simulink model "LongLatDriveline"  (R2024b)
settings: Solver=FixedStepAuto  StartTime=0  StopTime=120  FixedStep=0.002  RelTol=1e-3
InitFcn:
  | load('waypoints.mat');
  | VehicleObj = Simulink.data.dictionary.open('./ModelData/VehicleData.sldd');
  | %dDataSectObj = getSection(myDictionaryObj,'Design Data');
StopFcn:
  | Plot_LateralModelErrorControl;
  | 
  | mdlWks = get_param(gcs, 'ModelWorkspace');
  | par_ToDrvDesigner = evalin(mdlWks, 'ToDrvDesigner');
  | 
  | if par_ToDrvDesigner.Value
  |     ExportdrivingScenario;
  | end
model workspace (MAT data in the model file):
  ToDrvDesigner : Simulink.Parameter (value not decoded)
values from neighbouring files (symbols this model uses):
  A_F = 2.341157    [VehicleData.sldd]
  C_af = 80000.0    [VehicleData.sldd]
  C_ar = 80000.0    [VehicleData.sldd]
  C_d = 0.24    [VehicleData.sldd]
  f = 0.01    [VehicleData.sldd]
  g = 9.81    [VehicleData.sldd]
  h_aero = 0.65    [VehicleData.sldd]
  h_gc = 0.65    [VehicleData.sldd]
  Iz = 2873.0    [VehicleData.sldd]
  lf = 1.1    [VehicleData.sldd]
  lr = 1.58    [VehicleData.sldd]
  m = 2238.932    [VehicleData.sldd]
  Nf = 2.0    [VehicleData.sldd]
  Nr = 2.0    [VehicleData.sldd]
  r_stat = 0.342    [VehicleData.sldd]
  r_w = 0.352    [VehicleData.sldd]
  rho = 1.225    [VehicleData.sldd]
  theta = 0.0    [VehicleData.sldd]
  transGear = 0.1027    [VehicleData.sldd]
  V_wind = 0.0    [VehicleData.sldd]
symbols that are objects in the model workspace (value not decoded): ToDrvDesigner
undefined symbols (not defined in the file or in its folder): InitialPsi, InitialX, InitialY, phi
libraries: slpidlib x14, spsMosfetLib x6, simulink x4, spsVoltageMeasurementLib x3, SignalEditorBlockLib x2, spsDCVoltageSourceLib x1, spspowerguiLib x1
(part 4 of 5)

== matlab function LongLatDriveline/LateralController/HOSMC_AckermanSuperTwist/HOSMC_AckermanSuperTwis1 ==
  data: U output size=1; E input; Vx input; Mu1 input; C_af parameter; g parameter; C_ar parameter; lf parameter; lr parameter; Iz parameter; m parameter; dMu1 output
% ******************* Lateral dynamic controller *********************
%*********************************************************************
% Author: L.Arturo Torres-Romero
% Date: 22-10-2020
% This controller controlls the direction of a car, based in the dynamics
% described  in the next link and using the conventional sliding mode control 
% formulation with the procedure of converting to regular form: 
% https://www.researchgate.net/publication/340166902_LATERAL_VEHICLE_DYNAMICS_AND_CONTROLLERS_DESIGN
%******************* PARAMETERS DESCRIPTIONS **********************
%******************************************************************
% m: vehicle mass
% g: gravity
% C_af : Cornering  stiffness  of  front  wheels.
% C_ar : Cornering  stiffness  of  rear  wheels.
% lf : distance fron the center of gravity to the front wheel axis.
% lr : distance fron the center of gravity to the rear wheel axis.
% Iz : this is the momentum of inertia of the vehicle respect the z axis.
%******************************************************************
%******************* INPUTS DESCRIPTIONS **************************
%******************************************************************
% E:   (column vector)[e1;de1;e2;de2] states of the state space of 
%       the system that includes the errors as follows:
%      e1  : is the lateral position error respect the road.
%      de1 : derivative of e1.
%      e2  : is the yaw angle error with respect the road. 
%      de2 : derivarive of the e2.
% Vx: Logitudinal velocity.

%******************************************************************
% ******************* OUTPUTS DESCRIPTIONS ************************
%******************************************************************
% U: control coutput in radians. Angle of the frontal wheels respect to the
%    longitudinal axis
% isCtrl: when true means that the matrix Mc has full rank, and hence, the
%         system is controllable
%******************************************************************

function [U, dMu1] = SMC_AckermanSuperTwistingCtrl(E, Vx, Mu1,C_af, g, C_ar, lf, lr, Iz, m) % pd polos deseados
X = [0; 0; 0; 0];
X(1) = E(1);
X(2) = E(2);
X(3) = E(3);
X(4) = E(4);
%**************************************************
%******* Matrix A formulation *********************
A22 = -(2*C_af + 2*C_ar)/(m*Vx);
A23 = (2*C_af + 2*C_ar)/m;
A24 = (-2*C_af*lf + 2*C_ar*lr)/(m*Vx);
A42 = -(2*C_af*lf - 2*C_ar*lr)/(Iz*Vx);
A43 = (2*C_af*lf - 2*C_ar*lr)/Iz;
A44 = -(2*C_af*lf^2 + 2*C_ar*lr^2)/(Iz*Vx);

A = [0 1 0 0;0 A22 A23 A24;0 0 0 1;0 A42 A43 A44];
%**************************************************

%**************************************************
%******* Matrix B1 formulation ********************
B1_2 = 2*C_af/m;
B1_4 = 2*C_af*lf/Iz;

B1 = [0;B1_2;0;B1_4];
%***************************************************

%***************************************************
%******* Matrix B2 formulation *********************
B2_2 = -(2*C_af*lf - 2*C_ar*lr)/(m*Vx) - Vx;
B2_4 = -(2*C_af*lf^2 + 2*C_ar*lr^2)/(Iz*Vx);

B2 = [0;B2_2;0;B2_4];
%***************************************************


%***************************************************
%******* Matrix B3 formulation *********************
B3 = [0;g;0;0];
%***************************************************


%***************************************************
%******* Verification of controllability and output 
% calculation of the controller
%**************************************************
d_k = 0;
Mc = [B1 A*B1 A^2*B1 A^3*B1];
rankVal = rank(Mc);
    if rankVal < size(A,1)
        %disp('Not completely state controllable');
        isCtrl = 0;
        d_k = 0;
    else
        %disp('Completely state controllable');
        isCtrl = 1;
        % Pole placement
        %Pd =[-5-3i -5+3i -7 -10];
        Pd =[-5-5i -5+5i -7 -10];

        H = (A- Pd(1)*eye(4)) * (A- Pd(2)*eye(4)) * (A- Pd(3)*eye(4)) * (A- Pd(4)*eye(4));

        %ackerman formula
        K = [0 0 0 1]*Mc^-1*H;
        d_k = -K*X;  
    end

%*********** Controller parameters **************
k_smc = 100;   %10
sigma = 40;    %60
gamma1 = 1;
gamma2 = 1;
gamma = [0 gamma1 0 gamma2];

h_c = gamma*[0;3;0;3];
g_c = gamma*B1;
q = 0.3;

UM = abs(h_c/g_c)/q;

%***********************************************
e_c = gamma*[0; X(1);0;X(3)];
d_u = (-1/(gamma*B1))*(sigma*sqrt(abs(e_c))*sign(e_c) + Mu1);

if abs(Mu1) > UM 
   dMu1 = -Mu1;
else
   dMu1 = -k_smc*sign(e_c); 
end

ctrlVal = d_k + d_u;

U = real(ctrlVal);

== matlab function LongLatDriveline/LateralController/SMC_ConventionalRegularForm ==
  data: U output size=1; E input; Vx input; dPsi_des input; C_af parameter; g parameter; C_ar parameter; lf parameter; lr parameter; Iz parameter; m parameter; phi_ref input

% ******************* Lateral dynamic controller *********************
%*********************************************************************
% Author: L.Arturo Torres-Romero
% Date: 22-10-2020
% This controller controlls the direction of a car, based in the dynamics
% described  in the next link and using the conventional sliding mode control 
% formulation with the procedure of converting to regular form: 
% https://www.researchgate.net/publication/340166902_LATERAL_VEHICLE_DYNAMICS_AND_CONTROLLERS_DESIGN
%******************* PARAMETERS DESCRIPTIONS **********************
%******************************************************************
% m: vehicle mass
% g: gravity
% C_af : Cornering  stiffness  of  front  wheels.
% C_ar : Cornering  stiffness  of  rear  wheels.
% lf : distance fron the center of gravity to the front wheel axis.
% lr : distance fron the center of gravity to the rear wheel axis.
% Iz : this is the momentum of inertia of the vehicle respect the z axis.
%******************************************************************
%******************* INPUTS DESCRIPTIONS **************************
%******************************************************************
% E:   (column vector)[e1;de1;e2;de2] states of the state space of 
%       the system that includes the errors as follows:
%      e1  : is the lateral position error respect the road.
%      de1 : derivative of e1.
%      e2  : is the yaw angle error with respect the road. 
%      de2 : derivarive of the e2.
% Vx: Logitudinal velocity.

%******************************************************************
% ******************* OUTPUTS DESCRIPTIONS ************************
%******************************************************************
% U: control coutput in radians. Angle of the frontal wheels respect to the
%    longitudinal axis
% isCtrl: when true means that the matrix Mc has full rank, and hence, the
%         system is controllable
%******************************************************************

function U = SMC_ConventionalCtr2(E, Vx, dPsi_des,C_af, g, C_ar, lf, lr, Iz, m, phi_ref) % pd polos deseados
J = [0; 0; 0; 0];
J(1) = E(3);
J(2) = E(4);
J(3) = E(1);
J(4) = E(2);
phi = phi_ref;
%**************************************************
%******* Matrix A formulation *********************
A22 = -(2*C_af + 2*C_ar)/(m*Vx);
A23 = (2*C_af + 2*C_ar)/m;
A24 = (-2*C_af*lf + 2*C_ar*lr)/(m*Vx);
A42 = -(2*C_af*lf - 2*C_ar*lr)/(Iz*Vx);
A43 = (2*C_af*lf - 2*C_ar*lr)/Iz;
A44 = -(2*C_af*lf^2 + 2*C_ar*lr^2)/(Iz*Vx);

%A = [0 1 0 0;0 A22 A23 A24;0 0 0 1;0 A42 A43 A44];
A = [0 0 0 1;0 A42 A43 A44;0 1 0 0;0 A22 A23 A24];

%**************************************************

%**************************************************
%******* Matrix B1 formulation ********************
B1_2 = 2*C_af/m;
B1_4 = 2*C_af*lf/Iz;

%B1 = [0;B1_2;0;B1_4];
B1 = [0;B1_4;0;B1_2];
%***************************************************

%***************************************************
%******* Matrix B2 formulation *********************
B2_2 = -(2*C_af*lf - 2*C_ar*lr)/(m*Vx) - Vx;
B2_4 = -(2*C_af*lf^2 + 2*C_ar*lr^2)/(Iz*Vx);

B2 = [0;B2_4;0;B2_2];
%***************************************************


%***************************************************
%******* Matrix B3 formulation *********************
B3 = [0;g;0;0];
%***************************************************

l1 = (A24 - Vx)*dPsi_des +g*sin(phi);
l2 = A44*dPsi_des;
L = [0;l2;0;l1];

C = [B1 A*B1 A^2*B1 A^3*B1]; % controllability matrix
Cinv = inv(C);
q = Cinv(4,:);
P = [q;q*A;q*A^2;q*A^3];
Tr = P;

X = Tr*J;

%%%%%%%%%%%%%%%%%%%%%%%%%%%%% SMC settings %%%%%%%%%%%%%%%%%%%%%%%%%%%%%%%
n1 = 140000;
lambda_1 = -2;
lambda_2 = -7;
lambda_3 = -3;

S = [(1000000*lambda_1*lambda_2*lambda_3)/(A23*B1_4 - A43*B1_2), (1000000*(A23^2*B1_4^3 + A43^2*B1_2^2*B1_4 + A22*A23*A24*B1_4^3 - A42*A43*A44*B1_2^3 - 2*A23*A43*B1_2*B1_4^2 - A43*A44*B1_2^3*lambda_1 - A43*A44*B1_2^3*lambda_2 - A43*A44*B1_2^3*lambda_3 - A22*A23*A44*B1_2*B1_4^2 - A22*A24*A43*B1_2*B1_4^2 - A23*A24*A42*B1_2*B1_4^2 + A22*A43*A44*B1_2^2*B1_4 + A23*A42*A44*B1_2^2*B1_4 + A24*A42*A43*B1_2^2*B1_4 - A23*A24*B1_2*B1_4^2*lambda_1 - A23*A24*B1_2*B1_4^2*lambda_2 - A23*A24*B1_2*B1_4^2*lambda_3 + A23*A44*B1_2^2*B1_4*lambda_1 + A24*A43*B1_2^2*B1_4*lambda_1 + A23*A44*B1_2^2*B1_4*lambda_2 + A24*A43*B1_2^2*B1_4*lambda_2 + A23*A44*B1_2^2*B1_4*lambda_3 + A24*A43*B1_2^2*B1_4*lambda_3 - A23*B1_2*B1_4^2*lambda_1*lambda_2 - A23*B1_2*B1_4^2*lambda_1*lambda_3 - A23*B1_2*B1_4^2*lambda_2*lambda_3 + A43*B1_2^2*B1_4*lambda_1*lambda_2 + A43*B1_2^2*B1_4*lambda_1*lambda_3 + A43*B1_2^2*B1_4*lambda_2*lambda_3 - A44*B1_2^3*lambda_1*lambda_2*lambda_3 + A22*B1_2*B1_4^2*lambda_1*lambda_2*lambda_3 + A24*B1_2^2*B1_4*lambda_1*lambda_2*lambda_3 - A42*B1_2^2*B1_4*lambda_1*lambda_2*lambda_3))/((A23*B1_4 - A43*B1_2)*(A24^2*B1_2*B1_4^2 - 2*A24*A44*B1_2^2*B1_4 - A42*A24*B1_2*B1_4^2 + A22*A24*B1_4^3 + A44^2*B1_2^3 + A42*A44*B1_2^2*B1_4 - A22*A44*B1_2*B1_4^2 - A43*B1_2*B1_4^2 + A23*B1_4^3)), (1000000*(A23^2*B1_4^3*lambda_1 + A23^2*B1_4^3*lambda_2 + A23^2*B1_4^3*lambda_3 + A23^2*A24*B1_4^3 - A43^2*A44*B1_2^3 + A24*A43^2*B1_2^2*B1_4 - A23^2*A44*B1_2*B1_4^2 + A43^2*B1_2^2*B1_4*lambda_1 + A43^2*B1_2^2*B1_4*lambda_2 + A43^2*B1_2^2*B1_4*lambda_3 - 2*A23*A24*A43*B1_2*B1_4^2 + 2*A23*A43*A44*B1_2^2*B1_4 - 2*A23*A43*B1_2*B1_4^2*lambda_1 - 2*A23*A43*B1_2*B1_4^2*lambda_2 - 2*A23*A43*B1_2*B1_4^2*lambda_3 - A22*A23*B1_4^3*lambda_1*lambda_2 - A22*A23*B1_4^3*lambda_1*lambda_3 - A22*A23*B1_4^3*lambda_2*lambda_3 - A43*A44*B1_2^3*lambda_1*lambda_2 - A43*A44*B1_2^3*lambda_1*lambda_3 - A43*A44*B1_2^3*lambda_2*lambda_3 + A22^2*B1_4^3*lambda_1*lambda_2*lambda_3 + A42^2*B1_2^2*B1_4*lambda_1*lambda_2*lambda_3 - A23*A24*B1_2*B1_4^2*lambda_1*lambda_2 - A23*A24*B1_2*B1_4^2*lambda_1*lambda_3 - A23*A24*B1_2*B1_4^2*lambda_2*lambda_3 + A22*A43*B1_2*B1_4^2*lambda_1*lambda_2 + A23*A42*B1_2*B1_4^2*lambda_1*lambda_2 + A22*A43*B1_2*B1_4^2*lambda_1*lambda_3 + A23*A42*B1_2*B1_4^2*lambda_1*lambda_3 + A22*A43*B1_2*B1_4^2*lambda_2*lambda_3 + A23*A42*B1_2*B1_4^2*lambda_2*lambda_3 + A23*A44*B1_2^2*B1_4*lambda_1*lambda_2 + A24*A43*B1_2^2*B1_4*lambda_1*lambda_2 + A23*A44*B1_2^2*B1_4*lambda_1*lambda_3 + A24*A43*B1_2^2*B1_4*lambda_1*lambda_3 + A23*A44*B1_2^2*B1_4*lambda_2*lambda_3 + A24*A43*B1_2^2*B1_4*lambda_2*lambda_3 - A42*A43*B1_2^2*B1_4*lambda_1*lambda_2 - A42*A43*B1_2^2*B1_4*lambda_1*lambda_3 - A42*A43*B1_2^2*B1_4*lambda_2*lambda_3 + A42*A44*B1_2^3*lambda_1*lambda_2*lambda_3 - A23*B1_2*B1_4^2*lambda_1*lambda_2*lambda_3 + A43*B1_2^2*B1_4*lambda_1*lambda_2*lambda_3 + A22*A24*B1_2*B1_4^2*lambda_1*lambda_2*lambda_3 - 2*A22*A42*B1_2*B1_4^2*lambda_1*lambda_2*lambda_3 - A22*A44*B1_2^2*B1_4*lambda_1*lambda_2*lambda_3 - A24*A42*B1_2^2*B1_4*lambda_1*lambda_2*lambda_3))/((A23*B1_4 - A43*B1_2)*(A24^2*B1_2*B1_4^2 - 2*A24*A44*B1_2^2*B1_4 - A42*A24*B1_2*B1_4^2 + A22*A24*B1_4^3 + A44^2*B1_2^3 + A42*A44*B1_2^2*B1_4 - A22*A44*B1_2*B1_4^2 - A43*B1_2*B1_4^2 + A23*B1_4^3)), (1000000*(A23*A24^2*B1_4^3 - A43*A44^2*B1_2^3 + A23*B1_4^3*lambda_1*lambda_2 + A23*B1_4^3*lambda_1*lambda_3 + A23*B1_4^3*lambda_2*lambda_3 + A23*A44^2*B1_2^2*B1_4 - A24^2*A43*B1_2*B1_4^2 + A23*A24*B1_4^3*lambda_1 + A23*A24*B1_4^3*lambda_2 + A23*A24*B1_4^3*lambda_3 - 2*A23*A24*A44*B1_2*B1_4^2 + 2*A24*A43*A44*B1_2^2*B1_4 - A23*A44*B1_2*B1_4^2*lambda_1 - A24*A43*B1_2*B1_4^2*lambda_1 - A23*A44*B1_2*B1_4^2*lambda_2 - A24*A43*B1_2*B1_4^2*lambda_2 - A23*A44*B1_2*B1_4^2*lambda_3 - A24*A43*B1_2*B1_4^2*lambda_3 + A43*A44*B1_2^2*B1_4*lambda_1 + A43*A44*B1_2^2*B1_4*lambda_2 + A43*A44*B1_2^2*B1_4*lambda_3 - A43*B1_2*B1_4^2*lambda_1*lambda_2 - A43*B1_2*B1_4^2*lambda_1*lambda_3 - A43*B1_2*B1_4^2*lambda_2*lambda_3 - A22*B1_4^3*lambda_1*lambda_2*lambda_3 - A24*B1_2*B1_4^2*lambda_1*lambda_2*lambda_3 + A42*B1_2*B1_4^2*lambda_1*lambda_2*lambda_3 + A44*B1_2^2*B1_4*lambda_1*lambda_2*lambda_3))/((A23*B1_4 - A43*B1_2)*(A24^2*B1_2*B1_4^2 - 2*A24*A44*B1_2^2*B1_4 - A42*A24*B1_2*B1_4^2 + A22*A24*B1_4^3 + A44^2*B1_2^3 + A42*A44*B1_2^2*B1_4 - A22*A44*B1_2*B1_4^2 - A43*B1_2*B1_4^2 + A23*B1_4^3))];

%%%%%%%%%%%%%%%%%%%%%%%%%%%%%%%%%%%%%%%%%%%%%%%%%%%%%%%%%%%%%%%%%%%%%%%%%%%%

sigma1 = S*X;
ctrlVal = -(S*B1)\(n1*sign(sigma1)+ S*A*X +S*L);
U = real(ctrlVal);    



%*****************************************************************************
%******* Live script for help in calculus of the controller ************
% 
% format rational
% syms A B Q R Tr B1_2 B1_4 A22 A23 A24 A42 A43 A44 delta x1 x2 x3 x4 l1 l2
% 
% % X  = [x1;x2;x3;x4]
% % A  = [0 1 0 0;0 A22 A23 A24;0 0 0 1;0 A42 A43 A44]
% % B1 = [0;B1_2;0;B1_4]
% % L  = [0;l1;0;l2]
% 
% X  = [x3;x4;x1;x2]
% A  = [0 0 0 1;0 A42 A43 A44;0 1 0 0;0 A22 A23 A24]
% B1 = [0;B1_4;0;B1_2]
% L  = [0;l2;0;l1]
% 
% %%%%%%%%%%%%%%%% Transform (Tr) with ackerman form %%%%%%%%%%%%%%%%
% % C = [B1 A*B1 A^2*B1 A^3*B1] % controllability matrix
% % tmp1 = [0 0 0 1]/C;
% % Tr=[tmp1;tmp1*A;tmp1*A^2;tmp1*A^3] % state transformation
% % disp("tmp1")
% % size(tmp1)
% % disp("tmp1*A")
% % size(tmp1*A)
% % disp("tmp1*A^2")
% % size(tmp1*A^2)
% % disp("tmp1*A^3")
% % size(tmp1*A^3)
% % disp("C:")
% % size(C)
% % disp("tmp1:")
% % size(tmp1)
% % disp("Tr:")
% % size(Tr)
% %%%%%%%%%%%%%%%%%%%%%%%%%%%%%%%%%%%%%%%%%%%%%%%%%%%%%%%%%%%%%%%%%
% 
% %%%%%%%%%%%% Transform (Tr) with Utkin apprach %%%%%%%%%%%%%%%%%%
% % B_1 = [0;0;B1_4];
% % B_2 = B1_2;
% % 
% % a = eye(3)
% % b = -B_1*(B_2^(-1))
% % c = [0 0 0]
% % d = B_2^(-1)
% % 
% % Tr = [a b;c d];
% %%%%%%%%%%%%%%%%%%%%%%%%%%%%%%%%%%%%%%%%%%%%%%%%%%%%%%%%%%%%%%%%%%
% 
% 
% %%%%%%%%%%%%%%%% Transform (Tr) with linear system controller form %%%%%%%%%%%%%%%%
% C = [B1 A*B1 A^2*B1 A^3*B1] % controllability matrix
% Cinv = inv(C)
% q = Cinv(4,:)
% P = [q;q*A;q*A^2;q*A^3]
% Tr = P
% %%%%%%%%%%%%%%%%%%%%%%%%%%%%%%%%%%%%%%%%%%%%%%%%%%%%%%%%%%
% 
% A_ = simplify(Tr*A/Tr)
% B_ = simplify(Tr*B1)
% 
% A_11 = A_(1:3,1:3);
% A_12 = A_(1:3,4);
% 
% syms s1 s2 s3 lambda lambda_1 lambda_2 lambda_3 S2
% 
% %find paramters given eigenvalues
% S = [s1 s2 s3];
% eqeigen = det(lambda*eye(3) - (A_11 - A_12*S));
% eqeigen = simplify(eqeigen);
% eqeigen = collect(eqeigen,lambda);
% polyCoef = coeffs(eqeigen, lambda);
% polyCoef = fliplr(polyCoef)
% %%%%%%%%%%%%%%%
% % desired polinomial characteristic
% desiredPoly = (lambda + lambda_1)*(lambda + lambda_2)*(lambda + lambda_3);
% desiredPoly = collect(desiredPoly);
% desiredCoefs = coeffs(desiredPoly, lambda);
% desiredCoefs = fliplr(desiredCoefs)
% 
% eq1 = desiredCoefs(1) == polyCoef(1);
% eq2 = desiredCoefs(2) == polyCoef(2);
% eq3 = desiredCoefs(3) == polyCoef(3);
% eq4 = desiredCoefs(4) == polyCoef(4);
% 
% system1 = [eq2;eq3;eq4];
% sol = solve(system1,[s1 s2 s3]);
% S_ = [sol.s1 sol.s2 sol.s3]
% 
% %test eigen values:
% charEq1 = subs(eqeigen,s1,sol.s1);
% charEq2 = subs(charEq1,s2,sol.s2);
% charEq3 = subs(charEq2,s3,sol.s3)
% tf = isAlways(charEq3==desiredPoly)
% 
% S2 = 1000000;
% S = S2*[S_ 1]*Tr;
% %S = [S_ 1]*Tr;
% disp("!!!!!!!!surface S: ")
% simplify(S)
% 
% 
% syms n sigma1 x1 x2 x3 x4 u1 u2 n1 n2 
% X = [x1;x2;x3;x4];
% U = u1;
% 
% SIGMA = S*X;
% 
% % rewriting to the original forms %%%%%%%%%%%%%%%
% X  = [x1;x2;x3;x4]
% A  = [0 1 0 0;0 A22 A23 A24;0 0 0 1;0 A42 A43 A44]
% B1 = [0;B1_2;0;B1_4]
% %%%%%%%%%%%%%%%%%%%%%%%%%%%%%%%%%%%%%%%%%%%%%%%
% 
% 
% disp("!!!!! Sliding function sigma_1: ")
% Sigma_1 = simplify(SIGMA);
% Sigma_1 = collect(Sigma_1,[x1;x2;x3;x4])
% 
% eqsolution = -n1*sign(sigma1) == S*(A*X + B1*U +L);
% sol1 = solve(eqsolution,u1);
% 
% disp("!!!!! final control u: ")
% finalControl = simplify(sol1);
% finalControl = collect(finalControl,[x1;x2;x3;x4])
% 
% 
% U = -inv(S*B1)*(n1*sign(sigma1)+ S*A*X +S*L)
% 
% isAlways(finalControl==U)

== matlab function LongLatDriveline/Power Module/BLDC Motor/BLDC  SVPWM/Fases abc1 ==
  data: X input; Fabc output
function Fabc = fcn(X)
Fabc = [0;0;0];
    theta = mod(X(4),2*pi); %X(4)
    %theta = mod(X,2*pi);
    
    if (0<=theta)&&(theta<(pi/6))
        Fa = (6/pi)*theta;
    elseif ((pi/6)<=theta)&&(theta<(5*pi/6))
        Fa = 1;
    elseif ((5*pi/6<=theta))&&(theta<(7*pi/6))
        Fa = (6/pi)*(pi-theta);
    elseif ((7*pi/6)<=theta)&&(theta<(11*pi/6))
        Fa = -1;
    elseif ((11*pi/6)<=theta)&&(theta<(2*pi))
        Fa = (6/pi)*(theta-2*pi);
    else
        Fa = NaN;
    end
    
    if (0<=theta)&&(theta<(3*pi/6))
        Fb = -1;
    elseif ((3*pi/6)<=theta)&&(theta<(5*pi/6))
        Fb = (6/pi)*(theta-(2*pi)/3);
    elseif ((5*pi/6)<=theta)&&(theta<(9*pi/6))
        Fb = 1;
    elseif ((9*pi/6)<=theta)&&(theta<(11*pi/6))
        Fb = (6/pi)*(-theta+(5*pi)/3);
    elseif ((11*pi/6)<=theta)&&(theta<(2*pi))
        Fb = -1;
    else
        Fb = NaN;
    end
    
    if (0<=theta)&&(theta<(pi/6))
        Fc = 1;
    elseif ((pi/6)<=theta)&&(theta<(3*pi/6))
        Fc = (6/pi)*(pi/3-theta);
    elseif ((3*pi/6)<=theta)&&(theta<(7*pi/6))
        Fc = -1;
    elseif ((7*pi/6)<=theta)&&(theta<(9*pi/6))
        Fc = (6/pi)*(theta-(4*pi)/3);
    elseif ((9*pi/6)<=theta)&&(theta<(2*pi))
        Fc = 1;
    else
        Fc = NaN; 
    end
    
    
%     
     Fa = sin(theta);
     Fb = sin(theta - 2*pi/3);
     Fc = sin(theta + 2*pi/3);
    
    Fabc = [Fa;Fb;Fc];
end

== matlab function LongLatDriveline/LateralController/HOSMC_IntegralBlocksSuperTwisting/HOSMC_SuperTwisting ==
  data: U output size=1; d_k output; d_u output; E input; Vx input; dPsi_des input; phi_ref input; v input; e_bn input; C_af parameter; g parameter; C_ar parameter; lf parameter; lr parameter; Iz parameter; m parameter; dv output; de_bn output
% ******************* Lateral dynamic controller *********************

%*********************************************************************
% Author: L.Arturo Torres-Romero
% Date: 22-10-2025
% This controller controlls the direction of a car, based in the dynamics
% of the control by blocks with integral super-twisting SMC.
%  
% 
%******************* PARAMETERS DESCRIPTIONS **********************
%******************************************************************
% m: vehicle mass
% g: gravity
% C_af : Cornering  stiffness  of  front  wheels.
% C_ar : Cornering  stiffness  of  rear  wheels.
% lf : distance fron the center of gravity to the front wheel axis.
% lr : distance fron the center of gravity to the rear wheel axis.
% Iz : this is the momentum of inertia of the vehicle respect the z axis.
%******************************************************************
%******************* INPUTS DESCRIPTIONS **************************
%******************************************************************
% E:   (column vector)[e1;de1;e2;de2] states of the state space of 
%       the system that includes the errors as follows:
%      e1  : is the lateral position error respect the road.
%      de1 : derivative of e1.
%      e2  : is the yaw angle error with respect the road. 
%      de2 : derivarive of the e2.
% Vx: Logitudinal velocity.
% dPsi_des : Yaw derivative according the actual speed and road.
% phi_ref  : Superelevation of the road defined in the waipoints file. 
% v        : Integrated part of the STA.
% e_bn     : Nominal response of the error.
%******************************************************************
% ******************* OUTPUTS DESCRIPTIONS ************************
%******************************************************************
% U: control coutput in radians. Angle of the frontal wheels respect to the
%    longitudinal axis.
% d_k: Linear part of the control based on the known terms.
% d_u: Non linear part of the control bases on SMC super-twisting.
% dv : Switching part of the STA.
% de_bn: Dynamic of the nominal error.
%******************************************************************
function [U, d_k,d_u,dv,de_bn] = HOSMC_SuperTwistingCtrl...
    (E, Vx,dPsi_des, phi_ref, v,e_bn, C_af, g, C_ar, lf, lr, Iz, m) 
Y1 = [0;0];
Y2 = [0;0];

Y1 = [E(1);E(3)];
Y2 = [E(2);E(4)];
e = [E(2);E(3);E(4)];
%en = [Y2n(1); Y1n(2); Y2n(2)];
phi = phi_ref;

%**************************************************
%******* Matrix A formulation *********************
A22 = -(2*C_af + 2*C_ar)/(m*Vx);
A23 = (2*C_af + 2*C_ar)/m;
A24 = (-2*C_af*lf + 2*C_ar*lr)/(m*Vx);
A42 = -(2*C_af*lf - 2*C_ar*lr)/(Iz*Vx);
A43 = (2*C_af*lf - 2*C_ar*lr)/Iz;
A44 = -(2*C_af*lf^2 + 2*C_ar*lr^2)/(Iz*Vx);

A = [A22 A23 A24;A42 A43 A44];

%**************************************************
%******* Matrix B1 formulation ********************
B1_2 = 2*C_af/m;
B1_4 = 2*C_af*lf/Iz;

B1 = [B1_2;B1_4];
%***************************************************

%***************************************************
%******* Matrix L formulation *********************
l1 = (A24 - Vx)*dPsi_des +g*sin(phi);
l2 = A44*dPsi_des;
L = [l1;l2];

%***************************************************

%%
%%%%%%%%%%%%%% SUPER TWISTING 1 %%%%%%%%%%%%%%%%%
% %*********** Controller parameters **************
% k1 = 1;%6;      %7   18
% k2 = 15;%8;
%sigma = 10;    %60   10
gamma1 = 5;
gamma2 = 1;
gamma = [gamma1 gamma2];
%***************************************
h_c = abs(gamma*[0.8;0.4]);
g_c = abs(gamma*B1);
U_M = pi/8;

q = abs(h_c/g_c)/U_M;
C = abs(h_c);
k_v = C/(gamma*B1); %k_v = C/(gamma*B1) + 0.5;

k_u = sqrt(2/(gamma*B1*k_v - C));
k_u = k_u*(gamma*B1*k_v + C)*(1+q);
k_u = k_u/((gamma*B1)*(1-q)); %k_u = k_u/((gamma*B1)*(1-q)) + 0.8;


%*** Gains for s1 *******
k_v = 0.0065*1;
k_u = 0.0012*1.3;
%**********************


%***********************************************
k1 = 9;% 13.5
k2 = 8;% 5
e_b = -gamma*(k1*Y1+Y2);
d_k = -(1/(gamma*B1))*(gamma*(k1*Y2+A*e+L)-k2*e_b);

% dY2n = A*e + B1*d_k + L;
% dY1n = Y2n;


%************ two options for SMC surfaces *******
de_bn = -gamma*(k1*Y2 + A*e + B1*d_k + L);
s1 =  k2*(e_bn-e_b);


%***** the integration of dY1, dY2 must be implemented for this option
% e_t = gamma*(k1*Y1+Y2);     
% e_tn = gamma*(k1*Y1n+Y2n);
%s2 = e_t - e_tn; %(surface over the whole error of the states)
%*************************************************

s = s1;

d_u = -k_u*sqrt(abs(s))*sign(s) + v;

if abs(d_u) > U_M 
   dv = -d_u;
else
   dv = -k_v*sign(s); 
end

%%

%ctrlVal = d_k;
ctrlVal = d_k + d_u;
U = real(ctrlVal);

== matlab function LongLatDriveline/LateralController/HOSMC_RegularFormSuperTwist/HOSMC_RegularFormSuperTwist ==
  data: U output size=1; E input; Vx input; dPsi_des input; Mu1 input; C_af parameter; g parameter; C_ar parameter; lf parameter; lr parameter; Iz parameter; m parameter; dMu1 output; phi parameter
% ******************* Lateral dynamic controller *********************

%*********************************************************************
% Author: L.Arturo Torres-Romero
% Date: 22-10-2020
% This controller controlls the direction of a car, based in the dynamics
% described  in the next link and using the conventional sliding mode control 
% formulation with the procedure of converting to regular form: 
% https://www.researchgate.net/publication/340166902_LATERAL_VEHICLE_DYNAMICS_AND_CONTROLLERS_DESIGN
%******************* PARAMETERS DESCRIPTIONS **********************
%******************************************************************
% m: vehicle mass
% g: gravity
% C_af : Cornering  stiffness  of  front  wheels.
% C_ar : Cornering  stiffness  of  rear  wheels.
% lf : distance fron the center of gravity to the front wheel axis.
% lr : distance fron the center of gravity to the rear wheel axis.
% Iz : this is the momentum of inertia of the vehicle respect the z axis.
%******************************************************************
%******************* INPUTS DESCRIPTIONS **************************
%******************************************************************
% E:   (column vector)[e1;de1;e2;de2] states of the state space of 
%       the system that includes the errors as follows:
%      e1  : is the lateral position error respect the road.
%      de1 : derivative of e1.
%      e2  : is the yaw angle error with respect the road. 
%      de2 : derivarive of the e2.
% Vx: Logitudinal velocity.

%******************************************************************
% ******************* OUTPUTS DESCRIPTIONS ************************
%******************************************************************
% U: control coutput in radians. Angle of the frontal wheels respect to the
%    longitudinal axis
% isCtrl: when true means that the matrix Mc has full rank, and hence, the
%         system is controllable
%******************************************************************

function [U, dMu1] = HOSMC_RegularFormSuperTwistCtrl(E, Vx,dPsi_des, Mu1,C_af, g, C_ar, lf, lr, Iz, m,phi) % pd polos deseados
J = [0; 0; 0; 0];
J(1) = E(3);
J(2) = E(4);
J(3) = E(1);
J(4) = E(2);

%**************************************************
%******* Matrix A formulation *********************
A22 = -(2*C_af + 2*C_ar)/(m*Vx);
A23 = (2*C_af + 2*C_ar)/m;
A24 = (-2*C_af*lf + 2*C_ar*lr)/(m*Vx);
A42 = -(2*C_af*lf - 2*C_ar*lr)/(Iz*Vx);
A43 = (2*C_af*lf - 2*C_ar*lr)/Iz;
A44 = -(2*C_af*lf^2 + 2*C_ar*lr^2)/(Iz*Vx);

%A = [0 1 0 0;0 A22 A23 A24;0 0 0 1;0 A42 A43 A44];
A = [0 0 0 1;0 A42 A43 A44;0 1 0 0;0 A22 A23 A24];

%**************************************************

%**************************************************
%******* Matrix B1 formulation ********************
B1_2 = 2*C_af/m;
B1_4 = 2*C_af*lf/Iz;

%B1 = [0;B1_2;0;B1_4];
B1 = [0;B1_4;0;B1_2];
%***************************************************

%***************************************************
%******* Matrix B2 formulation *********************
B2_2 = -(2*C_af*lf - 2*C_ar*lr)/(m*Vx) - Vx;
B2_4 = -(2*C_af*lf^2 + 2*C_ar*lr^2)/(Iz*Vx);

B2 = [0;B2_4;0;B2_2];
%***************************************************


%***************************************************
%******* Matrix B3 formulation *********************
B3 = [0;g;0;0];
%***************************************************

l1 = (A24 - Vx)*dPsi_des +g*sin(phi);
l2 = A44*dPsi_des;
L = [0;l2;0;l1];

C = [B1 A*B1 A^2*B1 A^3*B1]; % controllability matrix
Cinv = inv(C);
q = Cinv(4,:);
P = [q;q*A;q*A^2;q*A^3];
Tr = P;

X = Tr*J;

%%%%%%%%%%%%%%%%%%%%%%%%%%%%% SMC settings %%%%%%%%%%%%%%%%%%%%%%%%%%%%%%%
n1 = 1;%140000;
lambda_1 = -2;
lambda_2 = -7;
lambda_3 = -3;

S = [(1000000*lambda_1*lambda_2*lambda_3)/(A23*B1_4 - A43*B1_2), (1000000*(A23^2*B1_4^3 + A43^2*B1_2^2*B1_4 + A22*A23*A24*B1_4^3 - A42*A43*A44*B1_2^3 - 2*A23*A43*B1_2*B1_4^2 - A43*A44*B1_2^3*lambda_1 - A43*A44*B1_2^3*lambda_2 - A43*A44*B1_2^3*lambda_3 - A22*A23*A44*B1_2*B1_4^2 - A22*A24*A43*B1_2*B1_4^2 - A23*A24*A42*B1_2*B1_4^2 + A22*A43*A44*B1_2^2*B1_4 + A23*A42*A44*B1_2^2*B1_4 + A24*A42*A43*B1_2^2*B1_4 - A23*A24*B1_2*B1_4^2*lambda_1 - A23*A24*B1_2*B1_4^2*lambda_2 - A23*A24*B1_2*B1_4^2*lambda_3 + A23*A44*B1_2^2*B1_4*lambda_1 + A24*A43*B1_2^2*B1_4*lambda_1 + A23*A44*B1_2^2*B1_4*lambda_2 + A24*A43*B1_2^2*B1_4*lambda_2 + A23*A44*B1_2^2*B1_4*lambda_3 + A24*A43*B1_2^2*B1_4*lambda_3 - A23*B1_2*B1_4^2*lambda_1*lambda_2 - A23*B1_2*B1_4^2*lambda_1*lambda_3 - A23*B1_2*B1_4^2*lambda_2*lambda_3 + A43*B1_2^2*B1_4*lambda_1*lambda_2 + A43*B1_2^2*B1_4*lambda_1*lambda_3 + A43*B1_2^2*B1_4*lambda_2*lambda_3 - A44*B1_2^3*lambda_1*lambda_2*lambda_3 + A22*B1_2*B1_4^2*lambda_1*lambda_2*lambda_3 + A24*B1_2^2*B1_4*lambda_1*lambda_2*lambda_3 - A42*B1_2^2*B1_4*lambda_1*lambda_2*lambda_3))/((A23*B1_4 - A43*B1_2)*(A24^2*B1_2*B1_4^2 - 2*A24*A44*B1_2^2*B1_4 - A42*A24*B1_2*B1_4^2 + A22*A24*B1_4^3 + A44^2*B1_2^3 + A42*A44*B1_2^2*B1_4 - A22*A44*B1_2*B1_4^2 - A43*B1_2*B1_4^2 + A23*B1_4^3)), (1000000*(A23^2*B1_4^3*lambda_1 + A23^2*B1_4^3*lambda_2 + A23^2*B1_4^3*lambda_3 + A23^2*A24*B1_4^3 - A43^2*A44*B1_2^3 + A24*A43^2*B1_2^2*B1_4 - A23^2*A44*B1_2*B1_4^2 + A43^2*B1_2^2*B1_4*lambda_1 + A43^2*B1_2^2*B1_4*lambda_2 + A43^2*B1_2^2*B1_4*lambda_3 - 2*A23*A24*A43*B1_2*B1_4^2 + 2*A23*A43*A44*B1_2^2*B1_4 - 2*A23*A43*B1_2*B1_4^2*lambda_1 - 2*A23*A43*B1_2*B1_4^2*lambda_2 - 2*A23*A43*B1_2*B1_4^2*lambda_3 - A22*A23*B1_4^3*lambda_1*lambda_2 - A22*A23*B1_4^3*lambda_1*lambda_3 - A22*A23*B1_4^3*lambda_2*lambda_3 - A43*A44*B1_2^3*lambda_1*lambda_2 - A43*A44*B1_2^3*lambda_1*lambda_3 - A43*A44*B1_2^3*lambda_2*lambda_3 + A22^2*B1_4^3*lambda_1*lambda_2*lambda_3 + A42^2*B1_2^2*B1_4*lambda_1*lambda_2*lambda_3 - A23*A24*B1_2*B1_4^2*lambda_1*lambda_2 - A23*A24*B1_2*B1_4^2*lambda_1*lambda_3 - A23*A24*B1_2*B1_4^2*lambda_2*lambda_3 + A22*A43*B1_2*B1_4^2*lambda_1*lambda_2 + A23*A42*B1_2*B1_4^2*lambda_1*lambda_2 + A22*A43*B1_2*B1_4^2*lambda_1*lambda_3 + A23*A42*B1_2*B1_4^2*lambda_1*lambda_3 + A22*A43*B1_2*B1_4^2*lambda_2*lambda_3 + A23*A42*B1_2*B1_4^2*lambda_2*lambda_3 + A23*A44*B1_2^2*B1_4*lambda_1*lambda_2 + A24*A43*B1_2^2*B1_4*lambda_1*lambda_2 + A23*A44*B1_2^2*B1_4*lambda_1*lambda_3 + A24*A43*B1_2^2*B1_4*lambda_1*lambda_3 + A23*A44*B1_2^2*B1_4*lambda_2*lambda_3 + A24*A43*B1_2^2*B1_4*lambda_2*lambda_3 - A42*A43*B1_2^2*B1_4*lambda_1*lambda_2 - A42*A43*B1_2^2*B1_4*lambda_1*lambda_3 - A42*A43*B1_2^2*B1_4*lambda_2*lambda_3 + A42*A44*B1_2^3*lambda_1*lambda_2*lambda_3 - A23*B1_2*B1_4^2*lambda_1*lambda_2*lambda_3 + A43*B1_2^2*B1_4*lambda_1*lambda_2*lambda_3 + A22*A24*B1_2*B1_4^2*lambda_1*lambda_2*lambda_3 - 2*A22*A42*B1_2*B1_4^2*lambda_1*lambda_2*lambda_3 - A22*A44*B1_2^2*B1_4*lambda_1*lambda_2*lambda_3 - A24*A42*B1_2^2*B1_4*lambda_1*lambda_2*lambda_3))/((A23*B1_4 - A43*B1_2)*(A24^2*B1_2*B1_4^2 - 2*A24*A44*B1_2^2*B1_4 - A42*A24*B1_2*B1_4^2 + A22*A24*B1_4^3 + A44^2*B1_2^3 + A42*A44*B1_2^2*B1_4 - A22*A44*B1_2*B1_4^2 - A43*B1_2*B1_4^2 + A23*B1_4^3)), (1000000*(A23*A24^2*B1_4^3 - A43*A44^2*B1_2^3 + A23*B1_4^3*lambda_1*lambda_2 + A23*B1_4^3*lambda_1*lambda_3 + A23*B1_4^3*lambda_2*lambda_3 + A23*A44^2*B1_2^2*B1_4 - A24^2*A43*B1_2*B1_4^2 + A23*A24*B1_4^3*lambda_1 + A23*A24*B1_4^3*lambda_2 + A23*A24*B1_4^3*lambda_3 - 2*A23*A24*A44*B1_2*B1_4^2 + 2*A24*A43*A44*B1_2^2*B1_4 - A23*A44*B1_2*B1_4^2*lambda_1 - A24*A43*B1_2*B1_4^2*lambda_1 - A23*A44*B1_2*B1_4^2*lambda_2 - A24*A43*B1_2*B1_4^2*lambda_2 - A23*A44*B1_2*B1_4^2*lambda_3 - A24*A43*B1_2*B1_4^2*lambda_3 + A43*A44*B1_2^2*B1_4*lambda_1 + A43*A44*B1_2^2*B1_4*lambda_2 + A43*A44*B1_2^2*B1_4*lambda_3 - A43*B1_2*B1_4^2*lambda_1*lambda_2 - A43*B1_2*B1_4^2*lambda_1*lambda_3 - A43*B1_2*B1_4^2*lambda_2*lambda_3 - A22*B1_4^3*lambda_1*lambda_2*lambda_3 - A24*B1_2*B1_4^2*lambda_1*lambda_2*lambda_3 + A42*B1_2*B1_4^2*lambda_1*lambda_2*lambda_3 + A44*B1_2^2*B1_4*lambda_1*lambda_2*lambda_3))/((A23*B1_4 - A43*B1_2)*(A24^2*B1_2*B1_4^2 - 2*A24*A44*B1_2^2*B1_4 - A42*A24*B1_2*B1_4^2 + A22*A24*B1_4^3 + A44^2*B1_2^3 + A42*A44*B1_2^2*B1_4 - A22*A44*B1_2*B1_4^2 - A43*B1_2*B1_4^2 + A23*B1_4^3))];

%%%%%%%%%%%%%%%%%%%%%%%%%%%%%%%%%%%%%%%%%%%%%%%%%%%%%%%%%%%%%%%%%%%%%%%%%%%%

k_smc = 1000*1.5;   %10
sigma = 6000*1.5;    %60

sigma1 = S*X;

d_k = -(S*B1)\(S*A*X +S*L);
d_u = -(S*B1)\(n1*sigma*sqrt(abs(sigma1))*sign(sigma1) + Mu1);
dMu1 = -k_smc*sign(sigma1); 

ctrlVal = d_k + d_u;
U = real(ctrlVal);

== matlab function LongLatDriveline/SteerActuator/BLDC_AngleCtrl/Back EMF ==
  data: X input; Fabc output
function Fabc = fcn(X)
Fabc = [0;0;0];
    theta = mod(X(5),2*pi); %X(4)
    %theta = mod(X,2*pi);
    
    if (0<=theta)&&(theta<(pi/6))
        Fa = (6/pi)*theta;
    elseif ((pi/6)<=theta)&&(theta<(5*pi/6))
        Fa = 1;
    elseif ((5*pi/6<=theta))&&(theta<(7*pi/6))
        Fa = (6/pi)*(pi-theta);
    elseif ((7*pi/6)<=theta)&&(theta<(11*pi/6))
        Fa = -1;
    elseif ((11*pi/6)<=theta)&&(theta<(2*pi))
        Fa = (6/pi)*(theta-2*pi);
    else
        Fa = NaN;
    end
    
    if (0<=theta)&&(theta<(3*pi/6))
        Fb = -1;
    elseif ((3*pi/6)<=theta)&&(theta<(5*pi/6))
        Fb = (6/pi)*(theta-(2*pi)/3);
    elseif ((5*pi/6)<=theta)&&(theta<(9*pi/6))
        Fb = 1;
    elseif ((9*pi/6)<=theta)&&(theta<(11*pi/6))
        Fb = (6/pi)*(-theta+(5*pi)/3);
    elseif ((11*pi/6)<=theta)&&(theta<(2*pi))
        Fb = -1;
    else
        Fb = NaN;
    end
    
    if (0<=theta)&&(theta<(pi/6))
        Fc = 1;
    elseif ((pi/6)<=theta)&&(theta<(3*pi/6))
        Fc = (6/pi)*(pi/3-theta);
    elseif ((3*pi/6)<=theta)&&(theta<(7*pi/6))
        Fc = -1;
    elseif ((7*pi/6)<=theta)&&(theta<(9*pi/6))
        Fc = (6/pi)*(theta-(4*pi)/3);
    elseif ((9*pi/6)<=theta)&&(theta<(2*pi))
        Fc = 1;
    else
        Fc = NaN; 
    end
    
    
%     
     %Fa = sin(theta);
     %Fb = sin(theta - 2*pi/3);
     %Fc = sin(theta + 2*pi/3);
    
    Fabc = [Fa;Fb;Fc];
end

== matlab function LongLatDriveline/Vehicle Lateral Model/DynamicModel/CoordConvertRotation/MATLAB Function ==
  data: A input; B output; theta input
function B = RotateVector(A, theta)
B = [0;0];
R = [cos(theta) -sin(theta); sin(theta) cos(theta)];

B = R*A;

== matlab function LongLatDriveline/Power Module/BLDC Motor/BLDC  SVPWM/Gráficas1 ==
  data: X input; theta output; Iabc output
function [theta,Iabc] = DEMUX(X)
theta = X(1);Iabc = X(2:4);

== matlab function LongLatDriveline/Vehicle Lateral Model/DynamicModel/LateralDynamics/LateralDynamic ==
  data: dX output; X input; Vx input; dd input; C_af parameter; C_ar parameter; lf parameter; lr parameter; Iz parameter; m parameter; g parameter; phi_ref input
% ******************* Lateral dynamic controller *********************
%*********************************************************************
% Author: L.Arturo Torres-Romero
% Date: 22-10-2020
% BICYCLE MODEL OF LATERAL VEHICLE DYNAMICS
% Based on Rajamani chapter 2.3 page 30 and  in the next publication with
% the controller
% https://www.researchgate.net/publication/340166902_LATERAL_VEHICLE_DYNAMICS_AND_CONTROLLERS_DESIGN
%******************* PARAMETERS DESCRIPTIONS **********************
%******************************************************************
% m: vehicle mass
% g: gravity
% C_af : Cornering  stiffness  of  front  wheels.
% C_ar : Cornering  stiffness  of  rear  wheels.
% lf : distance fron the center of gravity to the front wheel axis.
% lr : distance fron the center of gravity to the rear wheel axis.
% Iz : this is the momentum of inertia of the vehicle respect the z axis.
% phi : is the road bank. not used in this model.
%******************************************************************
%******************* INPUTS DESCRIPTIONS **************************
%******************************************************************
% X:   (column vector)[y;dy;Psi;dPsi] states of the state space of 
%       the system that includes:
%      y  : Radius of the curve that the car is performing.
%      dy : Lateral velocity.
%      Psi  : Is the yaw angle respect to the inertial global system
%      dPsi : Angular velocity of the yaw angle.
% Vx: Logitudinal velocity.

function dX = DynamicBicycleModel(X,Vx,dd, C_af, C_ar, lf, lr, Iz, m,g, phi_ref) % pd polos deseados
dX = [0;0;0;0];
y = X(1);
dy = X(2);
Psi = X(3);
dPsi = X(4);
phi = phi_ref;

A22 = -(2*C_af+2*C_ar)/(m*Vx);
A24 = -Vx- (2*C_af*lf-2*C_ar*lr)/(m*Vx);
A42 = -(2*lf*C_af-2*lr*C_ar)/(Iz*Vx);
A44 = -(2*lf^2*C_af + 2*lr^2*C_ar)/(Iz*Vx);

B21 = 2*C_af/m;
B41 = 2*lf*C_af/Iz;

A = [0 1 0 0;0 A22 0 A24;0 0 0 1;0 A42 0 A44];
B = [0;B21;0;B41];

dX= A*X(1:4) + B*dd; 

end

== matlab function LongLatDriveline/Vehicle Lateral Model/DynamicModel/LateralDynamics/LateralDynamic2 ==
  data: dX output; X input; Vx input; dd input; phi_ref input; C_af parameter; C_ar parameter; lf parameter; lr parameter; Iz parameter; m parameter; g parameter
% ******************* Lateral dynamic controller *********************
%*********************************************************************
% Author: L.Arturo Torres-Romero
% Date: 22-10-2020
% BICYCLE MODEL OF LATERAL VEHICLE DYNAMICS
% Based on Rajamani chapter 2.3 page 30 and  in the next publication with
% the controller
% https://www.researchgate.net/publication/340166902_LATERAL_VEHICLE_DYNAMICS_AND_CONTROLLERS_DESIGN
%******************* PARAMETERS DESCRIPTIONS **********************
%******************************************************************
% m: vehicle mass
% g: gravity
% C_af : Cornering  stiffness  of  front  wheels.
% C_ar : Cornering  stiffness  of  rear  wheels.
% lf : distance fron the center of gravity to the front wheel axis.
% lr : distance fron the center of gravity to the rear wheel axis.
% Iz : this is the momentum of inertia of the vehicle respect the z axis.
% phi: is the road bank.
%******************************************************************
%******************* INPUTS DESCRIPTIONS **************************
%******************************************************************
% X:   (column vector)[y;dy;Psi;dPsi] states of the state space of 
%       the system that includes:
%      y  : Radius of the curve that the car is performing.
%      dy : Lateral velocity.
%      Psi  : Is the yaw angle respect to the inertial global system
%      dPsi : Angular velocity of the yaw angle.
% Vx: Logitudinal velocity.

function dX = DynamicBicycleModel2(X,Vx,dd,phi_ref, C_af, C_ar, lf, lr, Iz, m,g) % pd polos deseados
dX = [0;0;0;0];
y = X(1);
dy = X(2);
Psi = X(3);
dPsi = X(4);

theta_vf = atan((dy + lf*dPsi)/Vx);
theta_vr = atan((dy - lr*dPsi)/Vx);

alpha_f = dd - theta_vf; % lateral slip angle in front tires
alpha_r = -theta_vr; % lateral slip angle in rear tires

dX(1) = X(2);
dX(2) = (2*C_af*alpha_f + 2*C_ar*alpha_r)/m + g*sin(phi_ref) - dPsi*Vx;
dX(3) = X(4);
dX(4) = (2*lf*C_af*alpha_f - 2*lr*C_ar*alpha_r)/Iz;

end

== matlab function LongLatDriveline/Vehicle Lateral Model/DynamicModel/LateralDynamics/LateralDynamicWithNoise/LateralDynamicWithNoise ==
  data: dX output; X input; Vx input; dd input; phi_ref input; NoiseDdy input; NoiseDdpsi input; C_af parameter; C_ar parameter; lf parameter; lr parameter; Iz parameter; m parameter; g parameter
% ******************* Lateral dynamic controller *********************
%*********************************************************************
% Author: L.Arturo Torres-Romero
% Date: 22-10-2020
% BICYCLE MODEL OF LATERAL VEHICLE DYNAMICS
% Based on Rajamani chapter 2.3 page 30 and  in the next publication with
% the controller
% https://www.researchgate.net/publication/340166902_LATERAL_VEHICLE_DYNAMICS_AND_CONTROLLERS_DESIGN
%******************* PARAMETERS DESCRIPTIONS **********************
%******************************************************************
% m: vehicle mass
% g: gravity
% C_af : Cornering  stiffness  of  front  wheels.
% C_ar : Cornering  stiffness  of  rear  wheels.
% lf : distance fron the center of gravity to the front wheel axis.
% lr : distance fron the center of gravity to the rear wheel axis.
% Iz : this is the momentum of inertia of the vehicle respect the z axis.
% phi: is the road bank.
%******************************************************************
%******************* INPUTS DESCRIPTIONS **************************
%******************************************************************
% X:   (column vector)[y;dy;Psi;dPsi] states of the state space of 
%       the system that includes:
%      y  : Radius of the curve that the car is performing.
%      dy : Lateral velocity.
%      Psi  : Is the yaw angle respect to the inertial global system
%      dPsi : Angular velocity of the yaw angle.
% Vx: Logitudinal velocity.

function dX = DynamicBicycleModel2(X,Vx,dd, phi_ref, NoiseDdy, NoiseDdpsi, C_af, C_ar, lf, lr, Iz, m,g) % pd polos deseados
dX = [0;0;0;0];
y = X(1);
dy = X(2);
Psi = X(3);
dPsi = X(4);
phi = phi_ref;

theta_vf = atan((dy + lf*dPsi)/Vx);
theta_vr = atan((dy - lr*dPsi)/Vx);

alpha_f = dd - theta_vf; % lateral slip angle in front tires
alpha_r = -theta_vr; % lateral slip angle in rear tires

dX(1) = X(2);
dX(2) = NoiseDdy + (2*C_af*alpha_f + 2*C_ar*alpha_r)/m + g*sin(phi) - dPsi*Vx;
dX(3) = X(4);
dX(4) = NoiseDdpsi + (2*lf*C_af*alpha_f - 2*lr*C_ar*alpha_r)/Iz;

end

== matlab function LongLatDriveline/Vehicle Lateral Model/DynamicModel/MATLAB Function ==
  data: u input; y output
function y = wrapTo2Pi(u)

y = wrapTo2Pi(u);

== matlab function LongLatDriveline/Vehicle Lateral Model/KinematicModel/LateralDynamic ==
  data: dX output; X input; Vx input; dd input; lf parameter; lr parameter; Iz parameter; m parameter; g parameter
% ******************* Lateral dynamic controller *********************
%*********************************************************************
% Author: L.Arturo Torres-Romero
% Date: 22-10-2020
% BICYCLE MODEL OF LATERAL VEHICLE DYNAMICS
% Based on Rajamani chapter 2.2 page 26
% 
%******************* PARAMETERS DESCRIPTIONS **********************
%******************************************************************
% m: vehicle mass
% g: gravity
% lf : distance fron the center of gravity to the front wheel axis.
% lr : distance fron the center of gravity to the rear wheel axis.
% Iz : this is the momentum of inertia of the vehicle respect the z axis.
% phi : is the road bank. not used in this model.
%******************************************************************
%******************* INPUTS DESCRIPTIONS **************************
%******************************************************************
% X:   (column vector)[y;dy;Psi;dPsi] states of the state space of 
%       the system that includes:
%      y  : Radius of the curve that the car is performing.
%      dy : Lateral velocity.
%      Psi  : Is the yaw angle respect to the inertial global system
%      dPsi : Angular velocity of the yaw angle.
% Vx: Logitudinal velocity.

function dX = KinematicBicycleModel(X,Vx,dd, lf, lr, Iz, m,g) % pd polos deseados
dX = [0;0;0];
y = X(1);
x = X(2);
Psi = X(3);

beta = atan((lr*tan(dd))/(lr+lf));
dPsi = (Vx*cos(beta))/(lr+lf)*tan(dd);
dx =   Vx*cos(beta+Psi);
dy =   Vx*sin(beta+Psi);

dX(1) = dy;
dX(2) = dx;
dX(3) = dPsi;

end

== matlab function LongLatDriveline/SteerActuator/BLDC_AngleCtrl/InvParkClarke ==
  data: X_dq input; Y_abc output; theta input
function Y_abc = fcn(X_dq, theta)
X_dq0 = [X_dq; 0];

%inverse Park-Clarke power invariant
iT_PC = sqrt(2/3)*[cos(theta)          -sin(theta)            1/sqrt(2); ...
                  cos(theta-2*pi/3)   -sin(theta-2*pi/3)     1/sqrt(2); ...
                  cos(theta+2*pi/3)   -sin(theta+2*pi/3)     1/sqrt(2)];
%               
              
 %inverse Park-Clarke amplitude invariant
% iT_PC = [cos(theta)          -sin(theta)            1; ...
%          cos(theta-2*pi/3)   -sin(theta-2*pi/3)     1; ...
%          cos(theta+2*pi/3)   -sin(theta+2*pi/3)     1];



Y_abc =iT_PC*X_dq0;
end
